simulink model "npc_controller"  (R2022a)
settings: Solver=FixedStepDiscrete  StartTime=0.0  StopTime=20  RelTol=1e-3  EnableMultiTasking=on
undefined symbols (not defined in the file): CAN_O_INT, CANA_BASE, Down, GPTRIP1SEL, GPTRIP2SEL, GPTRIP3SEL, Tsw, TZ1, TZ2, TZ3, Up, V2G_en
libraries: simulink x171, hdlsllib x90, c2802xlib x46, c2837xDlib x19, c280xlib x12, canmsglib x9, c2838xlib x8, idelinklib_common x5, c2806xlib x2, slpidlib x2, c28004xlib x2, c281xlib x2
(part 13 of 55)

== system npc_controller/IDLE_AND_TIMER/codegen/IDLE ==
  note: Note: GPIO6 J8.80
  note: Note: change to function call
  function : TriggerPort  TriggerType=function-call  VariantControl=Variant
  Function-Call Generator1 : simulink/Ports & Subsystems/Function-Call Generator  sample_time=-1  numberOfIterations=1  DisallowWideOutput=off
  Function-Call Split1 : FunctionCallSplit  NumOutputPorts=2
  Function-Call Split2 : FunctionCallSplit  NumOutputPorts=2
  Function-Call Split3 : FunctionCallSplit  NumOutputPorts=2
  GPIO6_HIGH : Subsystem  Commented=on
      settings: RTWSystemCode=Inline
  GPIO6_LOW : Subsystem  Commented=on
      settings: RTWSystemCode=Inline
  cnt_idle : Subsystem  TreatAsAtomicUnit=on
      settings: RTWSystemCode=Inline
  idle_task : Subsystem  TreatAsAtomicUnit=on
      settings: RTWSystemCode=Inline
  idle_task1 : Subsystem  Commented=on  TreatAsAtomicUnit=on
      settings: RTWSystemCode=Inline
  wires:
  Function-Call Split1/1 -> idle_task/Trigger
  Function-Call Split1/2 -> Function-Call Split2/1
  Function-Call Generator1/1 -> Function-Call Split3/1
  Function-Call Split3/1 -> GPIO6_HIGH/Trigger
  Function-Call Split3/2 -> Function-Call Split1/1
  Function-Call Split2/1 -> cnt_idle/Trigger
  Function-Call Split2/2 -> GPIO6_LOW/Trigger

== system npc_controller/IDLE_AND_TIMER/codegen/INITIALIZATION ==
  Function-Call Generator1 : simulink/Ports & Subsystems/Function-Call Generator  sample_time=-1  numberOfIterations=1  DisallowWideOutput=off
  Function-Call Split{1..3,5} (4 alike) : FunctionCallSplit  NumOutputPorts=2
  clb : Subsystem  Commented=on  TreatAsAtomicUnit=on
      settings: RTWSystemCode=Inline
  cmpss : Subsystem  TreatAsAtomicUnit=on
      settings: RTWSystemCode=Inline
  epwm : Subsystem  TreatAsAtomicUnit=on
      settings: RTWSystemCode=Inline
  epwm1 : Subsystem  Commented=on  TreatAsAtomicUnit=on
      settings: RTWSystemCode=Inline
  orps&relay : Subsystem  TreatAsAtomicUnit=on
      settings: RTWSystemCode=Inline
  outputxbar : Subsystem  Commented=on  TreatAsAtomicUnit=on
      settings: RTWSystemCode=Inline
  wires:
  Function-Call Generator1/1 -> Function-Call Split1/1
  Function-Call Split5/1 -> cmpss/Trigger
  Function-Call Split2/2 -> clb/Trigger
  Function-Call Split3/2 -> Function-Call Split5/1
  Function-Call Split2/1 -> outputxbar/Trigger
  Function-Call Split5/2 -> Function-Call Split2/1
  Function-Call Split3/1 -> orps&relay/Trigger
  Function-Call Split1/2 -> Function-Call Split3/1
  Function-Call Split1/1 -> epwm/Trigger

== system npc_controller/IDLE_AND_TIMER/codegen/TIMER_100MS ==
  note: Note: launchpad CANA, 32, 33
  note: Note:
      | Byte0 - func ID
      | Byte1 - MSB
      | Byte2 - LSB
  CAN Pack1 : canmsglib/CAN Pack  MsgList=(none)  MsgName=CAN Msg  MsgIDType=Standard (11-bit identifier)  MsgIdentifier=2  MsgLength=8  Remote=off  ApplyMinMax=off  BusOutput=off  SignalInfo={}
      settings: SourceProductBaseCode=ME,VN  DataFormat=raw data
  contstruct_can_msg : Subsystem
  eCAN Transmit : c280xlib/eCAN Transmit  chipFamily=C280x  useModule=eCAN_B  mailboxNo=1  messageID=bin2dec('111000111')  messageType=Standard (11-bit identifier)  enableBlockingMode=off  postInterrupt=off  interruptLine=0
      settings: SourceProductBaseCode=TIC2000
  get_func_id_data : Subsystem
  incr_cnt : Subsystem
  wires:
  CAN Pack1/1 -> eCAN Transmit/1
  contstruct_can_msg/1(can_msg) -> CAN Pack1/1
  get_func_id_data/2(data) -> contstruct_can_msg/2(data)
  get_func_id_data/1(func_id) -> contstruct_can_msg/1(func_id)

== system npc_controller/IDLE_AND_TIMER/codegen/TIMER_1MS ==
  note: 1) Add Subsystem or Model blocks as valid variant choices.
      | 2) You cannot connect blocks at this level. At simulation, connectivity is automatically
      | determined, based on the active variant and port name matching.
  codegen : Subsystem  VariantControl=sim_en==0
  sim : Subsystem  VariantControl=sim_en==1

== system npc_controller/IDLE_AND_TIMER/codegen/u32 Data to 2xu16 ==
  u32 Data : Inport
  Bit Shift : hdlsllib/Logic and Bit Operations/Bit Shift  mode=Shift Right Logical  N=8
  Bitwise AND : simulink/Logic and Bit Operations/Bitwise Operator  logicop=AND  UseBitMask=on  BitMask=bin2dec('00000000000000001111111111111111')  BitMaskRealWorld=Stored Integer
  Bitwise AND1 : simulink/Logic and Bit Operations/Bitwise Operator  logicop=AND  UseBitMask=on  BitMask=hex2dec('FFFF0000')  BitMaskRealWorld=Stored Integer
  Data Type Conversion : DataTypeConversion  OutDataTypeStr=uint16  SaturateOnIntegerOverflow=off  RndMeth=Floor
  Data Type Conversion1 : DataTypeConversion  OutDataTypeStr=uint16  SaturateOnIntegerOverflow=off  RndMeth=Floor
  u16Lsb : Outport
  u16Msb : Outport  Port=2
  wires:
  u32 Data/1 -> Bitwise AND1/1, Bitwise AND/1
  Bit Shift/1 -> Data Type Conversion1/1
  Bitwise AND/1 -> Data Type Conversion/1
  Data Type Conversion1/1 -> u16Msb/1
  Bitwise AND1/1 -> Bit Shift/1
  Data Type Conversion/1 -> u16Lsb/1

== system npc_controller/CONTROL/CONTROL/false/CLA_CONTROL ==
  va : Inport  OutDataTypeStr=single
  vb : Inport  Port=2  OutDataTypeStr=single
  vc : Inport  Port=3  OutDataTypeStr=single
  ia : Inport  Port=4  OutDataTypeStr=single
  ib : Inport  Port=5  OutDataTypeStr=single
  ic : Inport  Port=6  OutDataTypeStr=single
  vbulk : Inport  Port=7  OutDataTypeStr=single
  vmid : Inport  Port=8  OutDataTypeStr=single
  control_en : Inport  Port=9
  ref : Inport  Port=10
  angle : Inport  Port=11
  pol_pha : Inport  Port=12
  pol_phb : Inport  Port=13
  pol_phc : Inport  Port=14
  pha_en1 : Inport  Port=15
  phb_en1 : Inport  Port=16
  phc_en1 : Inport  Port=17
  pfc_ok2 : Inport  Port=18  OutDataTypeStr=boolean
  Trigger : TriggerPort  TriggerType=function-call  VariantControl=Variant  PortDimensions=1
  CONTROL : Subsystem
      settings: RTWSystemCode=Inline
  Function-Call Generator : simulink/Ports & Subsystems/Function-Call Generator  sample_time=-1  numberOfIterations=1  DisallowWideOutput=off
  Function-Call Split1 : FunctionCallSplit  NumOutputPorts=2
  Function-Call Split2 : FunctionCallSplit  NumOutputPorts=2
  Function-Call Split3 : FunctionCallSplit  NumOutputPorts=2
  GPIO_HIGH : Subsystem
      settings: RTWSystemCode=Inline
  GPIO_LOW : Subsystem
      settings: RTWSystemCode=Inline
  INIT/RESET_CONTROL : Subsystem
  sim_cmp : Outport
  Vpk : Outport  Port=2
  vbal_coef : Outport  Port=3
  wires:
  va/1 -> CONTROL/1(adc_out)  "cpu2cla_van"
  vb/1 -> CONTROL/2(adc_out1)  "cpu2cla_vbn"
  vc/1 -> CONTROL/3(adc_out2)  "cpu2cla_vcn"
  ia/1 -> CONTROL/4(adc_out3)  "cpu2cla_ia"
  ib/1 -> CONTROL/5(adc_out4)  "cpu2cla_ib"
  ic/1 -> CONTROL/6(adc_out5)  "cpu2cla_ic"
  vbulk/1 -> CONTROL/7(adc_out6)  "cpu2cla_vbulk"
  vmid/1 -> CONTROL/8(adc_out7)  "cpu2cla_vmid"
  ref/1 -> CONTROL/9(ref)  "cpu2cla_ref"
  Function-Call Split1/2 -> Function-Call Split3/1
  Function-Call Generator/1 -> Function-Call Split1/1
  Function-Call Split2/1 -> CONTROL/Trigger
  Function-Call Split2/2 -> GPIO_LOW/Trigger
  Function-Call Split1/1 -> GPIO_HIGH/Trigger
  CONTROL/1(sim_cmp) -> sim_cmp/1
  control_en/1 -> INIT/RESET_CONTROL/1(control_en)  "cpu2cla_control_en"
  Function-Call Split3/2 -> Function-Call Split2/1
  Function-Call Split3/1 -> INIT/RESET_CONTROL/Trigger
  pol_pha/1 -> CONTROL/11(pol_pha)  "cpu2cla_pol_pha"
  pol_phb/1 -> CONTROL/12(pol_phb)  "cpu2cla_pol_phb"
  pol_phc/1 -> CONTROL/13(pol_phc)  "cpu2cla_pol_phc"
  angle/1 -> CONTROL/10(angle)  "cpu2cla_angle"
  pha_en1/1 -> INIT/RESET_CONTROL/2(pha_en1)  "cpu2cla_pha_en"
  phb_en1/1 -> INIT/RESET_CONTROL/3(phb_en1)  "cpu2cla_phb_en"
  phc_en1/1 -> INIT/RESET_CONTROL/4(phc_en1)  "cpu2cla_phc_en"
  CONTROL/3(Vpk) -> Vpk/1  "cpu2cla_Vpk"
  pfc_ok2/1 -> CONTROL/14(pfc_ok2)  "cpu2cla_pfc_ok2"
  CONTROL/2(vbal_coef) -> vbal_coef/1  "cla2cpu_vbal_coef"

== system npc_controller/CONTROL/GET_ADC/ADC/codegen ==
  note: Note:
      | A0 VCSB_AD J3.30
      | A1 T_MUX_AD J7.70
      | A2 ICSC_AD J3.29
      | A3 VSCC_AD J3.26
      | A4 ICSA_AD J7.69
      | A5 VCSA_AD J7.66
      |
      | 14 ICSB_AD J3.23
      | 15 VBIAS_AD J7.63
      |
      | B0 IPHASE_A_ADC XX
      | B1 ADC_DEBUG_1 XX
      | B2 IPHASE_B_ADC J3.28
      | B3 IPHASE_C_ADC J3.25
      | B4 VPFC_OUT_AD J7.68
      | B5 VPFC_MID_AD J7.65
      |
      | *Near grid is ics
  adc_in : Inport
  3Ph Sine Gen : Subsystem  Commented=on
  ADCA : Subsystem
  ADCC : Subsystem
  Bus Creator1 : BusCreator  Inputs=8  OutDataTypeStr=Bus: adc
  Bus Creator2 : BusCreator  Inputs=8  OutDataTypeStr=Bus: adc_rect
  Constant : Constant  Commented=on  Value=2048  OutDataTypeStr=single  SampleTime=-1
  Data Store Read : DataStoreRead  Commented=on  DataStoreName=adc_vbulk  IndexOptions=Index vector (dialog)  Indices=1  OutputSizes=1
  Data Store Read1 : DataStoreRead  Commented=on  DataStoreName=adc_vmid  IndexOptions=Index vector (dialog)  Indices=1  OutputSizes=1
  Data Store Write7 : DataStoreWrite  Commented=on  DataStoreName=adc_vtop  IndexOptions=Index vector (dialog)  Indices=1  OutputSizes=1
  Function-Call Generator : simulink/Ports & Subsystems/Function-Call Generator  sample_time=-1  numberOfIterations=1  DisallowWideOutput=off
  Function-Call Split2 : FunctionCallSplit  NumOutputPorts=2
  Gain1 : Gain  Commented=on  Gain=2  ParamDataTypeStr=single  OutDataTypeStr=single
  Gain9 : Gain  Commented=on  Gain=2  ParamDataTypeStr=single  OutDataTypeStr=single
  IIR Filter7 : Subsystem  Commented=on
  Memory Copy : idelinklib_common/Memory Copy  Commented=on  copyFrom=Specified source code symbol  copyFromAddressSource=Specify via dialog  copyFromAddress=hex2dec('00001000')  copyFromSrcCode=&EPwm8Regs.CMPA.bit.CMPA  dataTypeFrom=uint16  dataDimensionFrom=1  useOffsetFrom=off  offsetFromSrc=Specify via dialog  offsetFrom=0  strideFrom=1  copyTo=Output port  copyToAddressSource=Specify via dialog  copyToAddress=hex2dec('00002000')  copyToSrcCode=myVariableDst  dataTypeTo=uint16  useOffsetTo=off  offsetToSrc=Specify via dialog  offsetTo=0  strideTo=1  sampleTime=inf  useInitValue=off  initValueSrc=Specify constant value  initValue=1  initValueSrcCode=myInitValueVariable  useAsMask=off  maskOperator=bitwise AND  useTermValue=off  termValue=1  isRealtimeEnabled=off  emitCCBeforeWrite=off  CCBeforeWrite=/* Custom Code Before Write*/  emitCCAfterWrite=off  CCAfterWrite=/* Custom Code After Write*/  useDMACopy=off  enableBlockingMode=off
      settings: SourceProductBaseCode=ME
  Memory Copy1 : idelinklib_common/Memory Copy  Commented=on  copyFrom=Specified source code symbol  copyFromAddressSource=Specify via dialog  copyFromAddress=hex2dec('00001000')  copyFromSrcCode=&EPwm2Regs.CMPB.bit.CMPB  dataTypeFrom=uint16  dataDimensionFrom=1  useOffsetFrom=off  offsetFromSrc=Specify via dialog  offsetFrom=0  strideFrom=1  copyTo=Output port  copyToAddressSource=Specify via dialog  copyToAddress=hex2dec('00002000')  copyToSrcCode=myVariableDst  dataTypeTo=uint16  useOffsetTo=off  offsetToSrc=Specify via dialog  offsetTo=0  strideTo=1  sampleTime=inf  useInitValue=off  initValueSrc=Specify constant value  initValue=1  initValueSrcCode=myInitValueVariable  useAsMask=off  maskOperator=bitwise AND  useTermValue=off  termValue=1  isRealtimeEnabled=off  emitCCBeforeWrite=off  CCBeforeWrite=/* Custom Code Before Write*/  emitCCAfterWrite=off  CCAfterWrite=/* Custom Code After Write*/  useDMACopy=off  enableBlockingMode=off
      settings: SourceProductBaseCode=ME
  Subsystem : Subsystem
  Subsystem1 : Subsystem
  Subsystem2 : Subsystem
  Subsystem3 : Subsystem
  Subsystem4 : Subsystem
  Subsystem5 : Subsystem
  Subsystem6 : Subsystem
  Subsystem7 : Subsystem
  Subsystem8 : Subsystem
  Subtract : Sum  Commented=on  Inputs=+-
  Sum : Sum  Commented=on  Inputs=|++
  adc_out : Outport
  adc_rect : Outport  Port=2
  wires:
  Data Store Read/1 -> Subtract/1
  Data Store Read1/1 -> Subtract/2
  Subtract/1 -> Data Store Write7/1
  [ic] -> Bus Creator1/6  "ic"
  [vmid] -> Bus Creator1/8  "vmid"
  [vbulk] -> Bus Creator1/7  "vbulk"
  Bus Creator1/1 -> adc_out/1  "vbulk"
  [ib] -> Bus Creator1/5  "ib"
  [ia] -> Bus Creator1/4  "ia"
  [ia] -> Subsystem3/1(adc)  "ia"
  [va] -> Subsystem/1(adc)  "va"
  [ic] -> Subsystem5/1(adc)  "ic"
  [vb] -> Subsystem1/1(adc)  "vb"
  [vmid] -> Bus Creator2/8  "vmid"
  [vc] -> Subsystem2/1(adc)  "vc"
  Subsystem5/1(adc_rect) -> Bus Creator2/6  "ic"
  [ib] -> Subsystem4/1(adc)  "ib"
  Subsystem4/1(adc_rect) -> Bus Creator2/5  "ib"
  Subsystem3/1(adc_rect) -> Bus Creator2/4  "ia"
  [vbulk] -> Bus Creator2/7  "vbulk"
  Bus Creator2/1 -> adc_rect/1
  Function-Call Split2/1 -> ADCA/Trigger
  Function-Call Generator/1 -> Function-Call Split2/1
  ADCA/1(vb) -> [vb]
  ADCA/4(ia) -> [ia]
  ADCA/3(vc) -> [vc]
  ADCA/2(ic) -> [ic]
  ADCA/5(va) -> [va]
  ADCA/6(ib) -> [ib]
  ADCC/4(vbulk) -> [vbulk]
  ADCC/5(vmid) -> [vmid]
  Function-Call Split2/2 -> ADCC/Trigger
  ADCC/3(iphasec) -> [iphasec]
  ADCC/2(iphaseb) -> [iphaseb]
  ADCC/1(iphasea) -> [iphasea]
  [iphasec] -> Subsystem8/1(adc)  "vc"
  [iphaseb] -> Subsystem7/1(adc)  "vb"
  [iphasea] -> Subsystem6/1(adc)  "va"
  3Ph Sine Gen/2(sine_b) -> Sum/1  "vb"
  Memory Copy/1 -> Gain9/1
  Gain9/1 -> ?
  Memory Copy1/1 -> Gain1/1
  Gain1/1 -> ?
  Sum/1 -> ?
  Constant/1 -> Sum/2
  [va] -> Bus Creator1/1  "va"
  [vb] -> Bus Creator1/2  "vb"
  [vc] -> Bus Creator1/3  "vc"
  Subsystem/1(adc_rect) -> Bus Creator2/1  "va"
  Subsystem1/1(adc_rect) -> Bus Creator2/2  "vb"
  Subsystem2/1(adc_rect) -> Bus Creator2/3  "vc"

== system npc_controller/CONTROL/GET_ADC/ADC/sim ==
  note: Notes:
      | vac_adc = vac_actual*0.00264706+1.65
      | iac_adc = iac_actual*0.02+1.65
      | vbulk_adc = vbulk_actual*3.49e-3
      | vmid_adc = vmid_acutal*3.49e-3
  note: Note:
      | Vmid         C2
      | Vbulk        A5
      |
      | Va            A2/B6
      | Vb            B0
      | Vc            C0
      |
      | Ia             A3
      | Ib             A10/B1, C10
      | Ic             C1
  note: since the current sense in hardware is -ve
  adc_in : Inport
  Bus Creator1 : BusCreator  Inputs=8  OutDataTypeStr=Bus: adc
  Bus Creator2 : BusCreator  Inputs=8  OutDataTypeStr=Bus: adc_rect
  Cast To Single : DataTypeConversion  OutDataTypeStr=single  SaturateOnIntegerOverflow=off  RndMeth=Floor
  Cast To Single1 : DataTypeConversion  OutDataTypeStr=single  SaturateOnIntegerOverflow=off  RndMeth=Floor
  Data Store Read : DataStoreRead  DataStoreName=adc_offset_vc  IndexOptions=Index vector (dialog)  Indices=1  OutputSizes=1
  Data Store Read1 : DataStoreRead  DataStoreName=adc_offset_ic  IndexOptions=Index vector (dialog)  Indices=1  OutputSizes=1
  Data Store Read2 : DataStoreRead  DataStoreName=adc_offset_vb  IndexOptions=Index vector (dialog)  Indices=1  OutputSizes=1
  Data Store Read4 : DataStoreRead  DataStoreName=adc_offset_va  IndexOptions=Index vector (dialog)  Indices=1  OutputSizes=1
  Data Store Read6 : DataStoreRead  DataStoreName=adc_offset_ia  IndexOptions=Index vector (dialog)  Indices=1  OutputSizes=1
  Data Store Read7 : DataStoreRead  DataStoreName=adc_offset_ib  IndexOptions=Index vector (dialog)  Indices=1  OutputSizes=1
  Demux : Demux  Outputs=8
  IIR Filter3 : Subsystem  Commented=on
  IIR Filter5 : Subsystem  Commented=on
  IIR Filter8 : Subsystem  Commented=on
  Scope2 : Scope
  Scope3 : Scope
  Subsystem : Subsystem
  Subsystem1 : Subsystem
  Subsystem2 : Subsystem
  Subsystem3 : Subsystem
  Subsystem4 : Subsystem
  Subsystem5 : Subsystem
  vabc{1..6} (6 alike) : Sum  Inputs=|+-  AccumDataTypeStr=single  OutDataTypeStr=single
  adc_out : Outport
  adc_rect : Outport  Port=2
  wires:
  adc_in/1 -> Demux/1
  Demux/7 -> Cast To Single/1
  Data Store Read6/1 -> vabc2/2
  Demux/4 -> vabc2/1
  vabc2/1 -> [ia]
  Bus Creator1/1 -> adc_out/1  "vbulk"
  Demux/6 -> vabc6/1
  Data Store Read2/1 -> vabc1/2
  Data Store Read1/1 -> Scope3/1, vabc6/2
  Data Store Read7/1 -> vabc5/2
  Demux/5 -> vabc5/1
  Demux/2 -> vabc1/1
  vabc3/1 -> [va]
  Data Store Read/1 -> Scope2/1, vabc4/2
  Data Store Read4/1 -> vabc3/2
  vabc1/1 -> [vb]
  vabc5/1 -> [ib]
  Demux/3 -> vabc4/1
  Demux/1 -> vabc3/1  "va"
  Demux/8 -> Cast To Single1/1  "vmid"
  [vb] -> Bus Creator1/2  "vb"
  [vc] -> Bus Creator1/3  "vc"
  [ia] -> Bus Creator1/4  "ia"
  [ib] -> Bus Creator1/5  "ib"
  [ic] -> Bus Creator1/6  "ic"
  [va] -> Bus Creator1/1  "va"
  [vbulk] -> Bus Creator1/7  "vbulk"
  [vmid] -> Bus Creator1/8  "vmid"
  Subsystem/1(adc_rect) -> Bus Creator2/1  "va"
  Subsystem1/1(adc_rect) -> Bus Creator2/2  "vb"
  Subsystem3/1(adc_rect) -> Bus Creator2/4  "ia"
  Subsystem4/1(adc_rect) -> Bus Creator2/5  "ib"
  Bus Creator2/1 -> adc_rect/1  "vbulk"
  [va] -> Subsystem/1(adc)  "va"
  [vb] -> Subsystem1/1(adc)  "vb"
  [vc] -> Subsystem2/1(adc)  "vc"
  [ia] -> Subsystem3/1(adc)  "ia"
  [ib] -> Subsystem4/1(adc)  "ib"
  [ic] -> Subsystem5/1(adc)  "ic"
  [vmid] -> Bus Creator2/8  "vmid"
  [vbulk] -> Bus Creator2/7  "vbulk"
  Subsystem2/1(adc_rect) -> Bus Creator2/3  "vc"
  Subsystem5/1(adc_rect) -> Bus Creator2/6  "ic"
  vabc4/1 -> [vc]  "va"
  vabc6/1 -> [ic]  "va"
  Cast To Single/1 -> [vbulk]
  Cast To Single1/1 -> [vmid]

== system npc_controller/CONTROL/POLARITY/PLL_Block1/SRF_PLL ==
  Vabc : Inport
  Demux1 : Demux  Outputs=3
  Gain : Gain  Commented=on  Gain=1/(2*pi)
  Integrator : Subsystem
  Memory : Memory  InheritSampleTime=on  LinearizeAsDelay=on
  PI : Subsystem
  Subsystem1 : Subsystem  Commented=on
  Sum1 : Sum  Inputs=|++  AccumDataTypeStr=single  OutDataTypeStr=single
  abc to dq : Subsystem
  f0 : Constant  Value=2*pi*50  OutDataTypeStr=fixdt('single', 'DataTypeOverride', 'Off')
  SinVal : Outport  VectorParamsAs1DForOutWhenUnconnected=off
  CosVal : Outport  Port=2  VectorParamsAs1DForOutWhenUnconnected=off
  theta : Outport  Port=3  OutDataTypeStr=single  VectorParamsAs1DForOutWhenUnconnected=off
  wires:
  Vabc/1 -> Demux1/1
  Memory/1 -> abc to dq/4(wt)
  Integrator/1(wt) -> Memory/1, theta/1
  abc to dq/1(q) -> PI/1(Vq)
  f0/1 -> Sum1/2
  Gain/1 -> Subsystem1/1(x[n])  "Freq_Unf"
  PI/1(PI Out) -> Sum1/1
  Sum1/1 -> Gain/1, Integrator/1(PI Out)
  Demux1/1 -> abc to dq/1(a)
  Demux1/2 -> abc to dq/2(b)
  Demux1/3 -> abc to dq/3(c)

== system npc_controller/CONTROL/POLARITY/PLL_Block1/Subsystem ==
  In1 : Inport
  Cast To Single : DataTypeConversion  OutDataTypeStr=single  SaturateOnIntegerOverflow=off  RndMeth=Floor
  Constant2 : Constant  Value=0
  GreaterThan1 : RelationalOperator  Operator=>  OutDataTypeStr=boolean  RndMeth=Simplest  InputSameDT=off
  Initialize at Zero Crossing : Subsystem  TreatAsAtomicUnit=on
  Out1 : Outport
  wires:
  GreaterThan1/1 -> Initialize at Zero Crossing/Trigger, Initialize at Zero Crossing/1(In1)
  Constant2/1 -> GreaterThan1/2
  Initialize at Zero Crossing/1(Out1) -> Cast To Single/1
  In1/1 -> GreaterThan1/1
  Cast To Single/1 -> Out1/1

== system npc_controller/CONTROL/STATE-MACHINE/CPU_CONTROL_100_A2_precharge_pfc_ok2/configFutDis/System Outputs1 ==

== system npc_controller/CONTROL/STATE-MACHINE/CPU_CONTROL_100_A2_precharge_pfc_ok2/configFutDis/System Outputs2 ==

== system npc_controller/CONTROL/STATE-MACHINE/CPU_CONTROL_100_A2_precharge_pfc_ok2/configFutEn/System Outputs1 ==

== system npc_controller/CONTROL/STATE-MACHINE/CPU_CONTROL_100_A2_precharge_pfc_ok2/configFutEn/System Outputs2 ==

== system npc_controller/CONTROL/STATE-MACHINE/CPU_CONTROL_100_A2_precharge_pfc_ok2/configFutEn/System Outputs3 ==

== system npc_controller/CONTROL/STATE-MACHINE/CPU_CONTROL_100_A2_precharge_pfc_ok2/configGrid/FORCE_TZ ==
  note: 0 - Three phase
      | 1 - Single phase
  In1 : Inport
  sinlgeph_config : Inport  Port=2
  Trigger : TriggerPort  TriggerType=function-call  VariantControl=(inherit)  PortDimensions=1
  1P : Subsystem  TreatAsAtomicUnit=on
  3P3W : Subsystem  TreatAsAtomicUnit=on
  If : If  IfExpression=u1 == 0
  wires:
  If/1 -> 3P3W/Action
  sinlgeph_config/1 -> 1P/1(sinlgeph_config)
  If/2 -> 1P/Action
  In1/1 -> If/1

== system npc_controller/CONTROL/STATE-MACHINE/CPU_CONTROL_100_A2_precharge_pfc_ok2/configGrid/RESET_TZ ==
  note: EALLOW;
      |
      | /*Disabled tripzone action*/
      | EPwm6Regs.TZCTL.bit.TZA = (uint16_T)(0b11); //do nothing
      | EPwm6Regs.TZCTL.bit.TZB = (uint16_T)(0b11);
      | EPwm7Regs.TZCTL.bit.TZA = (uint16_T)(0b11);
      | EPwm7Regs.TZCTL.bit.TZB = (uint16_T)(0b11);
      | EPwm8Regs.TZCTL.bit.TZA = (uint16_T)(0b11);
      | EPwm8Regs.TZCTL.bit.TZB = (uint16_T)(0b11);
      | EPwm9Regs.TZCTL.bit.TZA = (uint16_T)(0b11);
      | EPwm9Regs.TZCTL.bit.TZB = (uint16_T)(0b11);
      | EPwm10Regs.TZCTL.bit.TZA = (uint16_T)(0b11);
      | EPwm10Regs.TZCTL.bit.TZB = (uint16_T)(0b11);
      | EPwm11Regs.TZCTL.bit.TZA = (uint16_T)(0b11);
      | EPwm11Regs.TZCTL.bit.TZB = (uint16_T)(0b11);
      |
      | /*Clear grouped OST TZ flags*/
      | EPwm6Regs.TZCLR.bit.OST = 0b1; //clear trip
      | EPwm7Regs.TZCLR.bit.OST = 0b1;
      | EPwm8Regs.TZCLR.bit.OST = 0b1;
      | EPwm9Regs.TZCLR.bit.OST = 0b1;
      | EPwm10Regs.TZCLR.bit.OST = 0b1;
      | EPwm11Regs.TZCLR.bit.OST = 0b1;
      |
      | /*Clear individual OST TZ flags*/
      | EPwm6Regs.TZOSTCLR.bit.OST1 = 0b1; //clear trip
      | EPwm6Regs.TZOSTCLR.bit.OST2 = 0b1;
      | EPwm7Regs.TZOSTCLR.bit.OST1 = 0b1;
      | EPwm7Regs.TZOSTCLR.bit.OST2 = 0b1;
      | EPwm8Regs.TZOSTCLR.bit.OST1 = 0b1;
      | EPwm8Regs.TZOSTCLR.bit.OST2 = 0b1;
      | EPwm9Regs.TZOSTCLR.bit.OST1 = 0b1;
      | EPwm9Regs.TZOSTCLR.bit.OST2 = 0b1;
      | EPwm10Regs.TZOSTCLR.bit.OST1 = 0b1;
      | EPwm10Regs.TZOSTCLR.bit.OST2 = 0b1;
      | EPwm11Regs.TZOSTCLR.bit.OST1 = 0b1;
      | EPwm11Regs.TZOSTCLR.bit.OST2 = 0b1;
      |
      | /*Enable tripzone action*/
      | EPwm6Regs.TZCTL.bit.TZA = (uint16_T)(0b10); //force to LOW
      | EPwm6Regs.TZCTL.bit.TZB = (uint16_T)(0b10);
      | EPwm7Regs.TZCTL.bit.TZA = (uint16_T)(0b10);
      | EPwm7Regs.TZCTL.bit.TZB = (uint16_T)(0b10);
      | EPwm8Regs.TZCTL.bit.TZA = (uint16_T)(0b10);
      | EPwm8Regs.TZCTL.bit.TZB = (uint16_T)(0b10);
      | EPwm9Regs.TZCTL.bit.TZA = (uint16_T)(0b10);
      | EPwm9Regs.TZCTL.bit.TZB = (uint16_T)(0b10);
      | EPwm10Regs.TZCTL.bit.TZA = (uint16_T)(0b10);
      | EPwm10Regs.TZCTL.bit.TZB = (uint16_T)(0b10);
      | EPwm11Regs.TZCTL.bit.TZA = (uint16_T)(0b10);
      | EPwm11Regs.TZCTL.bit.TZB = (uint16_T)(0b10);
      |
      | EDIS;
  note: Note:
      | TZCCTL
      | 0b00 - High impedance
      | 0b01 - Force to HIGH
      | 0b10 - Force to LOW
      | 0b11 - Do nothing
      |
      | AQCSFRC
      | 0b00 - disables forced PWM
      | 0b01 - forces PWM to LOW
      | 0b10 - forces PWM to  HIGH
      |
      | TZFRC.bit.OST
      | 0b0 - Do nothing
      | 0b1 - Force TZ
  Trigger : TriggerPort  TriggerType=function-call  VariantControl=(inherit)  PortDimensions=1
  System Outputs2 : Subsystem  mask(System Outputs){ShowInLibBrowser=0}
      mask prompts: ShowInLibBrowser "Simulink:masks:CustCodeMaskParam1_MP"
      settings: CopyFcn=cccopyfcn(gcb)  OpenFcn=ccopenfcn('System Outputs Function')
      mask Help: eval('feval(''rtwprivate'',''rtwhelpview'',''rtw_sys_outputs_block'')');
      mask Display: disp('System\nOutputs');

== system npc_controller/CONTROL/STATE-MACHINE/CPU_CONTROL_100_A2_precharge_pfc_ok2/detectPOSPhB/pos ==
  note: Note:
      | AQCSFRC
      | 0b00 - disables forced PWM
      | 0b01 - forces PWM to LOW
      | 0b10 - forces PWM to  HIGH
  note: Note:
      |
      | Function PWM # GPIO # LAUNCHPAD PIN #
      |
      | Synci EPWM1A GPIO0 J4.40
      | EPWM1B GPIO1 J4.39
      |
      | TZ GPIO62 XX
      |
      | a_s1 EPWM6B GPIO11 J8.75
      | a_s2 EPWM7B GPIO13 XX
      | a_s3 EPWM6A GPIO10 J8.76
      | a_s4 EPWM7A GPIO12 XX
      |
      | b_s1 EPWM8B GPIO15 J8.73
      | b_s2 EPWM9B GPIO17 XX
      | b_s3 EPWM8A GPIO14 J8.74
      | b_s4 EPWM9A GPIO16 J4.33
      |
      | c_s1 EPWM10B GPIO19 J1.3
      | c_s2 EPWM11B GPIO21 XX
      | c_s3 EPWM10A GPIO18 J1.4
      | c_s4 EPWM11A GPIO20 XX
  note: EPwm8Regs.AQCSFRC.bit.CSFB = (uint16_T)(0b01);
      | EPwm9Regs.AQCSFRC.bit.CSFB = (uint16_T)(0b10);
      | EPwm8Regs.AQCSFRC.bit.CSFA = (uint16_T)(0b00);
      | EPwm9Regs.AQCSFRC.bit.CSFA = (uint16_T)(0b01);
  Action Port : ActionPort  ActionPortLabel=elseif(u1 >= 16)
  Constant : Constant  OutDataTypeStr=uint8  SampleTime=-1
  System Outputs1 : Subsystem  mask(System Outputs){ShowInLibBrowser=0}
      mask prompts: ShowInLibBrowser "Simulink:masks:CustCodeMaskParam1_MP"
      settings: CopyFcn=cccopyfcn(gcb)  OpenFcn=ccopenfcn('System Outputs Function')
      mask Help: eval('feval(''rtwprivate'',''rtwhelpview'',''rtw_sys_outputs_block'')');
      mask Display: disp('System\nOutputs');
  pos : Outport
  wires:
  Constant/1 -> pos/1

== system npc_controller/CONTROL/STATE-MACHINE/CPU_CONTROL_100_A2_precharge_pfc_ok2/detectUvpOvp1/False ==
  Action Port : ActionPort
  Constant : Constant  Value=0  OutDataTypeStr=boolean  SampleTime=-1
  low : Outport
  wires:
  Constant/1 -> low/1

== system npc_controller/CONTROL/STATE-MACHINE/CPU_CONTROL_100_A2_precharge_pfc_ok2/detectUvpOvp1/True ==
  Action Port : ActionPort
  Constant1 : Constant  OutDataTypeStr=boolean  SampleTime=-1
  high : Outport
  wires:
  Constant1/1 -> high/1

== system npc_controller/CONTROL/STATE-MACHINE/CPU_CONTROL_100_A2_precharge_pfc_ok2/detectZCPhA/false ==
  Action Port : ActionPort  ActionPortLabel=else
  Constant1 : Constant  Value=0  OutDataTypeStr=boolean  SampleTime=-1
  ph_en_out : Outport
  wires:
  Constant1/1 -> ph_en_out/1

== system npc_controller/CONTROL/STATE-MACHINE/CPU_CONTROL_100_A2_precharge_pfc_ok2/detectZCPhA/true ==
  Action Port : ActionPort  ActionPortLabel="if((u1 > -5)  & (u1 < 5))"
  Constant : Constant  OutDataTypeStr=boolean  SampleTime=-1
  ph_en : Outport
  wires:
  Constant/1 -> ph_en/1

== system npc_controller/CONTROL/STATE-MACHINE/CPU_CONTROL_100_A2_precharge_pfc_ok2/detectZCPhB/false ==
  Action Port : ActionPort  ActionPortLabel=else
  Constant1 : Constant  Value=0  OutDataTypeStr=boolean  SampleTime=-1
  ph_en_out : Outport
  wires:
  Constant1/1 -> ph_en_out/1

== system npc_controller/CONTROL/STATE-MACHINE/CPU_CONTROL_100_A2_precharge_pfc_ok2/detectZCPhB/true ==
  Action Port : ActionPort  ActionPortLabel="if((u1 > -5)  & (u1 < 5))"
  Constant : Constant  OutDataTypeStr=boolean  SampleTime=-1
  ph_en : Outport
  wires:
  Constant/1 -> ph_en/1

== system npc_controller/CONTROL/STATE-MACHINE/CPU_CONTROL_100_A2_precharge_pfc_ok2/detectZCPhC/false ==
  Action Port : ActionPort  ActionPortLabel=else
  Constant1 : Constant  Value=0  OutDataTypeStr=boolean  SampleTime=-1
  ph_en_out : Outport
  wires:
  Constant1/1 -> ph_en_out/1

== system npc_controller/CONTROL/STATE-MACHINE/CPU_CONTROL_100_A2_precharge_pfc_ok2/detectZCPhC/true ==
  Action Port : ActionPort  ActionPortLabel="if((u1 > -5)  & (u1 < 5))"
  Constant : Constant  OutDataTypeStr=boolean  SampleTime=-1
  ph_en : Outport
  wires:
  Constant/1 -> ph_en/1

== system npc_controller/CONTROL/STATE-MACHINE/CPU_CONTROL_100_A2_precharge_pfc_ok2/disDigCmpMode/System Outputs2 ==

== system npc_controller/CONTROL/STATE-MACHINE/CPU_CONTROL_100_A2_precharge_pfc_ok2/disablePwm/System Outputs ==

== system npc_controller/CONTROL/STATE-MACHINE/CPU_CONTROL_100_A2_precharge_pfc_ok2/enDigCmpMode/System Outputs2 ==

== system npc_controller/CONTROL/STATE-MACHINE/CPU_CONTROL_100_A2_precharge_pfc_ok2/updateCalib/cnt ==
  cnt_calib : Inport  OutDataTypeStr=uint16
  van : Inport  Port=2  OutDataTypeStr=single  PortDimensions=1
  vbn : Inport  Port=3  OutDataTypeStr=single  PortDimensions=1
  vcn : Inport  Port=4  OutDataTypeStr=single  PortDimensions=1
  ia : Inport  Port=5  OutDataTypeStr=single  PortDimensions=1
  ib : Inport  Port=6  OutDataTypeStr=single  PortDimensions=1
  ic : Inport  Port=7  OutDataTypeStr=single  PortDimensions=1
  Action Port : ActionPort  ActionPortLabel=else
  Add : Sum  AccumDataTypeStr=uint16  OutDataTypeStr=uint16
  Constant : Constant  OutDataTypeStr=uint16  SampleTime=-1
  Constant1 : Constant  Value=0  OutDataTypeStr=boolean  SampleTime=-1
  Data Store Write : DataStoreWrite  DataStoreName=adc_offset_ib_tmp  IndexOptions=Index vector (dialog)  Indices=1  OutputSizes=1
  Data Store Write1 : DataStoreWrite  DataStoreName=adc_offset_ic_tmp  IndexOptions=Index vector (dialog)  Indices=1  OutputSizes=1
  Data Store Write2 : DataStoreWrite  DataStoreName=cnt_calib  IndexOptions=Index vector (dialog)  Indices=1  OutputSizes=1
  Data Store Write3 : DataStoreWrite  DataStoreName=adc_offset_vc_tmp  IndexOptions=Index vector (dialog)  Indices=1  OutputSizes=1
  Data Store Write4 : DataStoreWrite  DataStoreName=adc_offset_ia_tmp  IndexOptions=Index vector (dialog)  Indices=1  OutputSizes=1
  Data Store Write5 : DataStoreWrite  DataStoreName=adc_offset_va_tmp  IndexOptions=Index vector (dialog)  Indices=1  OutputSizes=1
  Data Store Write6 : DataStoreWrite  DataStoreName=adc_offset_vb_tmp  IndexOptions=Index vector (dialog)  Indices=1  OutputSizes=1
  IIR Filter2 : Subsystem  Commented=on
  Subsystem1 : Subsystem
  Subsystem2 : Subsystem
  Subsystem3 : Subsystem
  Subsystem4 : Subsystem
  Subsystem5 : Subsystem
  Subsystem6 : Subsystem
  calib_ok : Outport
  wires:
  cnt_calib/1 -> Add/1
  Add/1 -> Data Store Write2/1
  Constant1/1 -> calib_ok/1
  Subsystem2/1(average) -> Data Store Write/1  "va"
  Constant/1 -> Add/2
  Subsystem1/1(average) -> Data Store Write1/1  "va"
  Subsystem3/1(average) -> Data Store Write4/1  "va"
  Subsystem4/1(average) -> Data Store Write3/1  "va"
  Subsystem6/1(average) -> Data Store Write5/1  "va"
  van/1 -> Subsystem6/1(sample)
  Subsystem5/1(average) -> Data Store Write6/1  "va"
  vcn/1 -> Subsystem4/1(sample)
  vbn/1 -> Subsystem5/1(sample)
  ia/1 -> Subsystem3/1(sample)
  ic/1 -> Subsystem1/1(sample)
  ib/1 -> Subsystem2/1(sample)

== system npc_controller/CONTROL/STATE-MACHINE/CPU_CONTROL_100_A2_precharge_pfc_ok2/updateCalib/done ==
  Action Port : ActionPort  ActionPortLabel=if(u1 > 65000)
  AUTO-CALIB_DONE : Subsystem
  CLEAR_FAULTS : Subsystem
  Function-Call Generator : simulink/Ports & Subsystems/Function-Call Generator  sample_time=-1  numberOfIterations=1  DisallowWideOutput=off
  Function-Call Split1 : FunctionCallSplit  NumOutputPorts=2
  Function-Call Split2 : FunctionCallSplit  NumOutputPorts=2
  RESET_TZ : Subsystem
  calib_ok : Outport
  wires:
  Function-Call Generator/1 -> Function-Call Split1/1
  Function-Call Split1/2 -> Function-Call Split2/1
  AUTO-CALIB_DONE/1(Out1) -> calib_ok/1
  Function-Call Split1/1 -> AUTO-CALIB_DONE/Trigger
  Function-Call Split2/1 -> RESET_TZ/Trigger
  Function-Call Split2/2 -> CLEAR_FAULTS/Trigger

== system npc_controller/CONTROL/STATE-MACHINE/CPU_CONTROL_100_A2_precharge_pfc_ok2/updatePll3p/PLL ==
  abc : Inport
  Demux : Demux  Commented=on  Outputs=3
  If1 : If  Commented=on  IfExpression=(u1 > 0)  ShowElse=off
  SRF_PLL : Subsystem
  Subsystem : Subsystem  Commented=on
  theta : Outport  OutDataTypeStr=single
  wires:
  SRF_PLL/3(theta) -> theta/1
  Subsystem/1(Out1) -> If1/1
  abc/1 -> SRF_PLL/1(Vabc), Demux/1
  Demux/1 -> Subsystem/1(In1)

== system npc_controller/CONTROL/STATE-MACHINE/CPU_CONTROL_100_A2_precharge_pfc_ok2/updateSequencePhA/pol_final1 ==
  vxn : Inport
  ix : Inport  Port=2
  Trigger : TriggerPort  TriggerType=function-call  VariantControl=(inherit)  PortDimensions=1
  If : If  NumInputs=2  IfExpression="((u1 == 1)  & (u2 == 2)) | ((u1 == 2)  & (u2 == 1))"
  Merge : Merge
  pol_vxn : Subsystem  TreatAsAtomicUnit=on
  prot : Subsystem  TreatAsAtomicUnit=on
  pol : Outport
  wires:
  ix/1 -> If/2
  vxn/1 -> pol_vxn/1(vxn), If/1
  Merge/1 -> pol/1
  If/2 -> pol_vxn/Action
  prot/1(Out1) -> Merge/1
  If/1 -> prot/Action
  pol_vxn/1(Out1) -> Merge/2

== system npc_controller/CONTROL/STATE-MACHINE/CPU_CONTROL_100_A2_precharge_pfc_ok2/updateSequencePhA/pol_ix1 ==
  note: 75dig -> 3iac
  ix : Inport
  Trigger : TriggerPort  TriggerType=function-call  VariantControl=(inherit)  PortDimensions=1
  If : If  IfExpression="(u1 > -8)  & (u1 < 8)"  ElseIfExpressions=u1 >= 8
  Merge : Merge  Inputs=3
  neg : Subsystem  TreatAsAtomicUnit=on
  pos : Subsystem  TreatAsAtomicUnit=on
  zero : Subsystem  TreatAsAtomicUnit=on
  pol_ix : Outport
  wires:
  ix/1 -> If/1
  If/1 -> zero/Action
  zero/1(Out1) -> Merge/1
  If/2 -> pos/Action
  If/3 -> neg/Action
  neg/1(Out1) -> Merge/3
  pos/1(Out1) -> Merge/2
  Merge/1 -> pol_ix/1

== system npc_controller/CONTROL/STATE-MACHINE/CPU_CONTROL_100_A2_precharge_pfc_ok2/updateSequencePhA/pol_vxn1 ==
  note: 16dig -> 5vac
  vxn : Inport
  Trigger : TriggerPort  TriggerType=function-call  VariantControl=(inherit)  PortDimensions=1
  If : If  IfExpression="(u1 > -16)  & (u1 < 16)"  ElseIfExpressions=u1 >= 16
  Merge : Merge  Inputs=3
  neg : Subsystem  TreatAsAtomicUnit=on
  pos : Subsystem  TreatAsAtomicUnit=on
  zero : Subsystem  TreatAsAtomicUnit=on
  pol_vxn : Outport
  wires:
  Merge/1 -> pol_vxn/1
  pos/1(Out1) -> Merge/2
  neg/1(Out1) -> Merge/3
  If/3 -> neg/Action
  If/2 -> pos/Action
  zero/1(Out1) -> Merge/1
  If/1 -> zero/Action
  vxn/1 -> If/1

== system npc_controller/CONTROL/STATE-MACHINE/CPU_CONTROL_100_A2_precharge_pfc_ok2/updateSequencePhB/pol_final1 ==
  vxn : Inport
  ix : Inport  Port=2
  Trigger : TriggerPort  TriggerType=function-call  VariantControl=(inherit)  PortDimensions=1
  If : If  NumInputs=2  IfExpression="((u1 == 1)  & (u2 == 2)) | ((u1 == 2)  & (u2 == 1))"
  Merge : Merge
  pol_vxn : Subsystem  TreatAsAtomicUnit=on
  prot : Subsystem  TreatAsAtomicUnit=on
  pol : Outport
  wires:
  ix/1 -> If/2
  vxn/1 -> pol_vxn/1(vxn), If/1
  Merge/1 -> pol/1
  If/2 -> pol_vxn/Action
  prot/1(Out1) -> Merge/1
  If/1 -> prot/Action
  pol_vxn/1(Out1) -> Merge/2

== system npc_controller/CONTROL/STATE-MACHINE/CPU_CONTROL_100_A2_precharge_pfc_ok2/updateSequencePhB/pol_ix1 ==
  note: 75dig -> 3iac
  ix : Inport
  Trigger : TriggerPort  TriggerType=function-call  VariantControl=(inherit)  PortDimensions=1
  If : If  IfExpression="(u1 > -8)  & (u1 < 8)"  ElseIfExpressions=u1 >= 8
  Merge : Merge  Inputs=3
  neg : Subsystem  TreatAsAtomicUnit=on
  pos : Subsystem  TreatAsAtomicUnit=on
  zero : Subsystem  TreatAsAtomicUnit=on
  pol_ix : Outport
  wires:
  ix/1 -> If/1
  If/1 -> zero/Action
  zero/1(Out1) -> Merge/1
  If/2 -> pos/Action
  If/3 -> neg/Action
  neg/1(Out1) -> Merge/3
  pos/1(Out1) -> Merge/2
  Merge/1 -> pol_ix/1

== system npc_controller/CONTROL/STATE-MACHINE/CPU_CONTROL_100_A2_precharge_pfc_ok2/updateSequencePhB/pol_vxn1 ==
  note: 16dig -> 5vac
  vxn : Inport
  Trigger : TriggerPort  TriggerType=function-call  VariantControl=(inherit)  PortDimensions=1
  If : If  IfExpression="(u1 > -16)  & (u1 < 16)"  ElseIfExpressions=u1 >= 16
  Merge : Merge  Inputs=3
  neg : Subsystem  TreatAsAtomicUnit=on
  pos : Subsystem  TreatAsAtomicUnit=on
  zero : Subsystem  TreatAsAtomicUnit=on
  pol_vxn : Outport
  wires:
  Merge/1 -> pol_vxn/1
  pos/1(Out1) -> Merge/2
  neg/1(Out1) -> Merge/3
  If/3 -> neg/Action
  If/2 -> pos/Action
  zero/1(Out1) -> Merge/1
  If/1 -> zero/Action
  vxn/1 -> If/1

== system npc_controller/CONTROL/STATE-MACHINE/CPU_CONTROL_100_A2_precharge_pfc_ok2/updateSequencePhC/pol_final1 ==
  vxn : Inport
  ix : Inport  Port=2
  Trigger : TriggerPort  TriggerType=function-call  VariantControl=(inherit)  PortDimensions=1
  If : If  NumInputs=2  IfExpression="((u1 == 1)  & (u2 == 2)) | ((u1 == 2)  & (u2 == 1))"
  Merge : Merge
  pol_vxn : Subsystem  TreatAsAtomicUnit=on
  prot : Subsystem  TreatAsAtomicUnit=on
  pol : Outport
  wires:
  ix/1 -> If/2
  vxn/1 -> pol_vxn/1(vxn), If/1
  Merge/1 -> pol/1
  If/2 -> pol_vxn/Action
  prot/1(Out1) -> Merge/1
  If/1 -> prot/Action
  pol_vxn/1(Out1) -> Merge/2

== system npc_controller/CONTROL/STATE-MACHINE/CPU_CONTROL_100_A2_precharge_pfc_ok2/updateSequencePhC/pol_ix1 ==
  note: 75dig -> 3iac
  ix : Inport
  Trigger : TriggerPort  TriggerType=function-call  VariantControl=(inherit)  PortDimensions=1
  If : If  IfExpression="(u1 > -8)  & (u1 < 8)"  ElseIfExpressions=u1 >= 8
  Merge : Merge  Inputs=3
  neg : Subsystem  TreatAsAtomicUnit=on
  pos : Subsystem  TreatAsAtomicUnit=on
  zero : Subsystem  TreatAsAtomicUnit=on
  pol_ix : Outport
  wires:
  ix/1 -> If/1
  If/1 -> zero/Action
  zero/1(Out1) -> Merge/1
  If/2 -> pos/Action
  If/3 -> neg/Action
  neg/1(Out1) -> Merge/3
  pos/1(Out1) -> Merge/2
  Merge/1 -> pol_ix/1

== system npc_controller/CONTROL/STATE-MACHINE/CPU_CONTROL_100_A2_precharge_pfc_ok2/updateSequencePhC/pol_vxn1 ==
  note: 16dig -> 5vac
  vxn : Inport
  Trigger : TriggerPort  TriggerType=function-call  VariantControl=(inherit)  PortDimensions=1
  If : If  IfExpression="(u1 > -16)  & (u1 < 16)"  ElseIfExpressions=u1 >= 16
  Merge : Merge  Inputs=3
  neg : Subsystem  TreatAsAtomicUnit=on
  pos : Subsystem  TreatAsAtomicUnit=on
  zero : Subsystem  TreatAsAtomicUnit=on
  pol_vxn : Outport
  wires:
  Merge/1 -> pol_vxn/1
  pos/1(Out1) -> Merge/2
  neg/1(Out1) -> Merge/3
  If/3 -> neg/Action
  If/2 -> pos/Action
  zero/1(Out1) -> Merge/1
  If/1 -> zero/Action
  vxn/1 -> If/1

== system npc_controller/CONTROL/STATE-MACHINE/CPU_CONTROL_100_inv/ClrCmpssTz/System Outputs1 ==

== system npc_controller/CONTROL/STATE-MACHINE/CPU_CONTROL_100_inv/ClrCmpssTz/System Outputs2 ==

== system npc_controller/CONTROL/STATE-MACHINE/CPU_CONTROL_100_inv/configFutDis/System Outputs1 ==

== system npc_controller/CONTROL/STATE-MACHINE/CPU_CONTROL_100_inv/configFutDis/System Outputs2 ==

== system npc_controller/CONTROL/STATE-MACHINE/CPU_CONTROL_100_inv/configFutEn/System Outputs1 ==

== system npc_controller/CONTROL/STATE-MACHINE/CPU_CONTROL_100_inv/configFutEn/System Outputs2 ==

== system npc_controller/CONTROL/STATE-MACHINE/CPU_CONTROL_100_inv/configFutEn/System Outputs3 ==

== system npc_controller/CONTROL/STATE-MACHINE/CPU_CONTROL_100_inv/configGrid/FORCE_TZ ==
  note: 0 - Three phase
      | 1 - Single phase
  In1 : Inport
  sinlgeph_config : Inport  Port=2
  Trigger : TriggerPort  TriggerType=function-call  VariantControl=(inherit)  PortDimensions=1
  1P : Subsystem  TreatAsAtomicUnit=on
  3P3W : Subsystem  TreatAsAtomicUnit=on
  If : If  IfExpression=u1 == 0
  wires:
  If/1 -> 3P3W/Action
  sinlgeph_config/1 -> 1P/1(sinlgeph_config)
  If/2 -> 1P/Action
  In1/1 -> If/1

== system npc_controller/CONTROL/STATE-MACHINE/CPU_CONTROL_100_inv/configGrid/RESET_TZ ==
  note: EALLOW;
      |
      | /*Disabled tripzone action*/
      | EPwm6Regs.TZCTL.bit.TZA = (uint16_T)(0b11); //do nothing
      | EPwm6Regs.TZCTL.bit.TZB = (uint16_T)(0b11);
      | EPwm7Regs.TZCTL.bit.TZA = (uint16_T)(0b11);
      | EPwm7Regs.TZCTL.bit.TZB = (uint16_T)(0b11);
      | EPwm8Regs.TZCTL.bit.TZA = (uint16_T)(0b11);
      | EPwm8Regs.TZCTL.bit.TZB = (uint16_T)(0b11);
      | EPwm9Regs.TZCTL.bit.TZA = (uint16_T)(0b11);
      | EPwm9Regs.TZCTL.bit.TZB = (uint16_T)(0b11);
      | EPwm10Regs.TZCTL.bit.TZA = (uint16_T)(0b11);
      | EPwm10Regs.TZCTL.bit.TZB = (uint16_T)(0b11);
      | EPwm11Regs.TZCTL.bit.TZA = (uint16_T)(0b11);
      | EPwm11Regs.TZCTL.bit.TZB = (uint16_T)(0b11);
      |
      | /*Clear grouped OST TZ flags*/
      | EPwm6Regs.TZCLR.bit.OST = 0b1; //clear trip
      | EPwm7Regs.TZCLR.bit.OST = 0b1;
      | EPwm8Regs.TZCLR.bit.OST = 0b1;
      | EPwm9Regs.TZCLR.bit.OST = 0b1;
      | EPwm10Regs.TZCLR.bit.OST = 0b1;
      | EPwm11Regs.TZCLR.bit.OST = 0b1;
      |
      | /*Clear individual OST TZ flags*/
      | EPwm6Regs.TZOSTCLR.bit.OST1 = 0b1; //clear trip
      | EPwm6Regs.TZOSTCLR.bit.OST2 = 0b1;
      | EPwm7Regs.TZOSTCLR.bit.OST1 = 0b1;
      | EPwm7Regs.TZOSTCLR.bit.OST2 = 0b1;
      | EPwm8Regs.TZOSTCLR.bit.OST1 = 0b1;
      | EPwm8Regs.TZOSTCLR.bit.OST2 = 0b1;
      | EPwm9Regs.TZOSTCLR.bit.OST1 = 0b1;
      | EPwm9Regs.TZOSTCLR.bit.OST2 = 0b1;
      | EPwm10Regs.TZOSTCLR.bit.OST1 = 0b1;
      | EPwm10Regs.TZOSTCLR.bit.OST2 = 0b1;
      | EPwm11Regs.TZOSTCLR.bit.OST1 = 0b1;
      | EPwm11Regs.TZOSTCLR.bit.OST2 = 0b1;
      |
      | /*Enable tripzone action*/
      | EPwm6Regs.TZCTL.bit.TZA = (uint16_T)(0b10); //force to LOW
      | EPwm6Regs.TZCTL.bit.TZB = (uint16_T)(0b10);
      | EPwm7Regs.TZCTL.bit.TZA = (uint16_T)(0b10);
      | EPwm7Regs.TZCTL.bit.TZB = (uint16_T)(0b10);
      | EPwm8Regs.TZCTL.bit.TZA = (uint16_T)(0b10);
      | EPwm8Regs.TZCTL.bit.TZB = (uint16_T)(0b10);
      | EPwm9Regs.TZCTL.bit.TZA = (uint16_T)(0b10);
      | EPwm9Regs.TZCTL.bit.TZB = (uint16_T)(0b10);
      | EPwm10Regs.TZCTL.bit.TZA = (uint16_T)(0b10);
      | EPwm10Regs.TZCTL.bit.TZB = (uint16_T)(0b10);
      | EPwm11Regs.TZCTL.bit.TZA = (uint16_T)(0b10);
      | EPwm11Regs.TZCTL.bit.TZB = (uint16_T)(0b10);
      |
      | EDIS;
  note: Note:
      | TZCCTL
      | 0b00 - High impedance
      | 0b01 - Force to HIGH
      | 0b10 - Force to LOW
      | 0b11 - Do nothing
      |
      | AQCSFRC
      | 0b00 - disables forced PWM
      | 0b01 - forces PWM to LOW
      | 0b10 - forces PWM to  HIGH
      |
      | TZFRC.bit.OST
      | 0b0 - Do nothing
      | 0b1 - Force TZ
  Trigger : TriggerPort  TriggerType=function-call  VariantControl=(inherit)  PortDimensions=1
  System Outputs2 : Subsystem  mask(System Outputs){ShowInLibBrowser=0}
      mask prompts: ShowInLibBrowser "Simulink:masks:CustCodeMaskParam1_MP"
      settings: CopyFcn=cccopyfcn(gcb)  OpenFcn=ccopenfcn('System Outputs Function')
      mask Help: eval('feval(''rtwprivate'',''rtwhelpview'',''rtw_sys_outputs_block'')');
      mask Display: disp('System\nOutputs');

== system npc_controller/CONTROL/STATE-MACHINE/CPU_CONTROL_100_inv/detectZCPhA/false ==
  Action Port : ActionPort
  Constant1 : Constant  Value=0  OutDataTypeStr=boolean  SampleTime=-1
  ph_en_out : Outport
  wires:
  Constant1/1 -> ph_en_out/1

== system npc_controller/CONTROL/STATE-MACHINE/CPU_CONTROL_100_inv/detectZCPhA/true ==
  Action Port : ActionPort
  Constant : Constant  OutDataTypeStr=boolean  SampleTime=-1
  ph_en : Outport
  wires:
  Constant/1 -> ph_en/1

== system npc_controller/CONTROL/STATE-MACHINE/CPU_CONTROL_100_inv/detectZCPhB/false ==
  Action Port : ActionPort
  Constant1 : Constant  Value=0  OutDataTypeStr=boolean  SampleTime=-1
  ph_en_out : Outport
  wires:
  Constant1/1 -> ph_en_out/1

== system npc_controller/CONTROL/STATE-MACHINE/CPU_CONTROL_100_inv/detectZCPhB/true ==
  Action Port : ActionPort
  Constant : Constant  OutDataTypeStr=boolean  SampleTime=-1
  ph_en : Outport
  wires:
  Constant/1 -> ph_en/1

== system npc_controller/CONTROL/STATE-MACHINE/CPU_CONTROL_100_inv/detectZCPhC/false ==
  Action Port : ActionPort
  Constant1 : Constant  Value=0  OutDataTypeStr=boolean  SampleTime=-1
  ph_en_out : Outport
  wires:
  Constant1/1 -> ph_en_out/1

== system npc_controller/CONTROL/STATE-MACHINE/CPU_CONTROL_100_inv/detectZCPhC/true ==
  Action Port : ActionPort
  Constant : Constant  OutDataTypeStr=boolean  SampleTime=-1
  ph_en : Outport
  wires:
  Constant/1 -> ph_en/1

== system npc_controller/CONTROL/STATE-MACHINE/CPU_CONTROL_100_inv/disCmpssTz/System Outputs1 ==

== system npc_controller/CONTROL/STATE-MACHINE/CPU_CONTROL_100_inv/disCmpssTz/System Outputs2 ==

== system npc_controller/CONTROL/STATE-MACHINE/CPU_CONTROL_100_inv/disablePwm/System Outputs ==

== system npc_controller/CONTROL/STATE-MACHINE/CPU_CONTROL_100_inv/readCmpssOcp/System Outputs1 ==

== system npc_controller/CONTROL/STATE-MACHINE/CPU_CONTROL_100_inv/updateCalib/cnt ==
  cnt_calib : Inport  OutDataTypeStr=uint16
  van : Inport  Port=2  OutDataTypeStr=single  PortDimensions=1
  vbn : Inport  Port=3  OutDataTypeStr=single  PortDimensions=1
  vcn : Inport  Port=4  OutDataTypeStr=single  PortDimensions=1
  ia : Inport  Port=5  OutDataTypeStr=single  PortDimensions=1
  ib : Inport  Port=6  OutDataTypeStr=single  PortDimensions=1
  ic : Inport  Port=7  OutDataTypeStr=single  PortDimensions=1
  Action Port : ActionPort
  Add : Sum  AccumDataTypeStr=uint16  OutDataTypeStr=uint16
  Constant : Constant  OutDataTypeStr=uint16  SampleTime=-1
  Constant1 : Constant  Value=0  OutDataTypeStr=boolean  SampleTime=-1
  Data Store Write : DataStoreWrite  DataStoreName=adc_offset_ib_tmp  IndexOptions=Index vector (dialog)  Indices=1  OutputSizes=1
  Data Store Write1 : DataStoreWrite  DataStoreName=adc_offset_ic_tmp  IndexOptions=Index vector (dialog)  Indices=1  OutputSizes=1
  Data Store Write2 : DataStoreWrite  DataStoreName=cnt_calib  IndexOptions=Index vector (dialog)  Indices=1  OutputSizes=1
  Data Store Write3 : DataStoreWrite  DataStoreName=adc_offset_vc_tmp  IndexOptions=Index vector (dialog)  Indices=1  OutputSizes=1
  Data Store Write4 : DataStoreWrite  DataStoreName=adc_offset_ia_tmp  IndexOptions=Index vector (dialog)  Indices=1  OutputSizes=1
  Data Store Write5 : DataStoreWrite  DataStoreName=adc_offset_va_tmp  IndexOptions=Index vector (dialog)  Indices=1  OutputSizes=1
  Data Store Write6 : DataStoreWrite  DataStoreName=adc_offset_vb_tmp  IndexOptions=Index vector (dialog)  Indices=1  OutputSizes=1
  IIR Filter2 : Subsystem  Commented=on
  Subsystem1 : Subsystem
  Subsystem2 : Subsystem
  Subsystem3 : Subsystem
  Subsystem4 : Subsystem
  Subsystem5 : Subsystem
  Subsystem6 : Subsystem
  calib_ok : Outport
  wires:
  cnt_calib/1 -> Add/1
  Add/1 -> Data Store Write2/1
  Constant1/1 -> calib_ok/1
  Subsystem2/1(average) -> Data Store Write/1  "va"
  Constant/1 -> Add/2
  Subsystem1/1(average) -> Data Store Write1/1  "va"
  Subsystem3/1(average) -> Data Store Write4/1  "va"
  Subsystem4/1(average) -> Data Store Write3/1  "va"
  Subsystem6/1(average) -> Data Store Write5/1  "va"
  van/1 -> Subsystem6/1(sample)
  Subsystem5/1(average) -> Data Store Write6/1  "va"
  vcn/1 -> Subsystem4/1(sample)
  vbn/1 -> Subsystem5/1(sample)
  ia/1 -> Subsystem3/1(sample)
  ic/1 -> Subsystem1/1(sample)
  ib/1 -> Subsystem2/1(sample)

== system npc_controller/CONTROL/STATE-MACHINE/CPU_CONTROL_100_inv/updateCalib/done ==
  Action Port : ActionPort
  AUTO-CALIB_DONE : Subsystem
  CLEAR_FAULTS : Subsystem
  Function-Call Generator : simulink/Ports & Subsystems/Function-Call Generator  sample_time=-1  numberOfIterations=1  DisallowWideOutput=off
  Function-Call Split1 : FunctionCallSplit  NumOutputPorts=2
  Function-Call Split2 : FunctionCallSplit  NumOutputPorts=2
  RESET_TZ : Subsystem
  calib_ok : Outport
  wires:
  Function-Call Generator/1 -> Function-Call Split1/1
  Function-Call Split1/2 -> Function-Call Split2/1
  AUTO-CALIB_DONE/1(Out1) -> calib_ok/1
  Function-Call Split1/1 -> AUTO-CALIB_DONE/Trigger
  Function-Call Split2/1 -> RESET_TZ/Trigger
  Function-Call Split2/2 -> CLEAR_FAULTS/Trigger

== system npc_controller/CONTROL/STATE-MACHINE/CPU_CONTROL_100_inv/updatePll3p/PLL ==
  abc : Inport
  Demux : Demux  Commented=on  Outputs=3
  If1 : If  Commented=on  IfExpression=(u1 > 0)  ShowElse=off
  SRF_PLL : Subsystem
  Subsystem : Subsystem  Commented=on
  theta : Outport  OutDataTypeStr=single
  wires:
  SRF_PLL/3(theta) -> theta/1
  Subsystem/1(Out1) -> If1/1
  abc/1 -> SRF_PLL/1(Vabc), Demux/1
  Demux/1 -> Subsystem/1(In1)

== system npc_controller/CONTROL/STATE-MACHINE/CPU_CONTROL_100_inv/updateSequencePhA/pol_final1 ==
  vxn : Inport
  ix : Inport  Port=2
  Trigger : TriggerPort  TriggerType=function-call  VariantControl=(inherit)  PortDimensions=1
  If : If  NumInputs=2  IfExpression="((u1 == 1)  & (u2 == 2)) | ((u1 == 2)  & (u2 == 1))"
  Merge : Merge
  pol_vxn : Subsystem  TreatAsAtomicUnit=on
  prot : Subsystem  TreatAsAtomicUnit=on
  pol : Outport
  wires:
  ix/1 -> If/2
  vxn/1 -> pol_vxn/1(vxn), If/1
  Merge/1 -> pol/1
  If/2 -> pol_vxn/Action
  prot/1(Out1) -> Merge/1
  If/1 -> prot/Action
  pol_vxn/1(Out1) -> Merge/2

== system npc_controller/CONTROL/STATE-MACHINE/CPU_CONTROL_100_inv/updateSequencePhA/pol_ix1 ==
  note: 75dig -> 3iac
  ix : Inport
  Trigger : TriggerPort  TriggerType=function-call  VariantControl=(inherit)  PortDimensions=1
  If : If  IfExpression="(u1 > -8)  & (u1 < 8)"  ElseIfExpressions=u1 >= 8
  Merge : Merge  Inputs=3
  neg : Subsystem  TreatAsAtomicUnit=on
  pos : Subsystem  TreatAsAtomicUnit=on
  zero : Subsystem  TreatAsAtomicUnit=on
  pol_ix : Outport
  wires:
  ix/1 -> If/1
  If/1 -> zero/Action
  zero/1(Out1) -> Merge/1
  If/2 -> pos/Action
  If/3 -> neg/Action
  neg/1(Out1) -> Merge/3
  pos/1(Out1) -> Merge/2
  Merge/1 -> pol_ix/1

== system npc_controller/CONTROL/STATE-MACHINE/CPU_CONTROL_100_inv/updateSequencePhA/pol_vxn1 ==
  note: 16dig -> 5vac
  vxn : Inport
  ixn1 : Inport  Port=2
  Trigger : TriggerPort  TriggerType=function-call  VariantControl=(inherit)  PortDimensions=1
  Constant1 : Constant  Commented=on  Value=2048  OutDataTypeStr=single  SampleTime=-1
  If : If  IfExpression="(u1 > -16)  & (u1 < 16)"  ElseIfExpressions=u1 >= 16
  Merge : Merge  Inputs=3
  Sum1 : Sum  Commented=on  Inputs=|++
  neg : Subsystem  TreatAsAtomicUnit=on
  pos : Subsystem  TreatAsAtomicUnit=on
  zero : Subsystem  TreatAsAtomicUnit=on
  pol_vxn : Outport
  wires:
  Constant1/1 -> Sum1/2
  Sum1/1 -> ?
  vxn/1 -> If/1, Sum1/1
  ixn1/1 -> pos/1(ixn), neg/1(ixn)
  Merge/1 -> pol_vxn/1
  pos/1(Out1) -> Merge/2
  neg/1(Out1) -> Merge/3
  If/3 -> neg/Action
  If/2 -> pos/Action
  zero/1(Out1) -> Merge/1
  If/1 -> zero/Action

== system npc_controller/CONTROL/STATE-MACHINE/CPU_CONTROL_100_inv/updateSequencePhA/pol_vxn2 ==
  note: 16dig -> 5vac
  vxn : Inport
  Trigger : TriggerPort  TriggerType=function-call  VariantControl=(inherit)  PortDimensions=1
  If : If  IfExpression="(u1 > -16)  & (u1 < 16)"  ElseIfExpressions=u1 >= 16
  Merge : Merge  Inputs=3
  neg : Subsystem  TreatAsAtomicUnit=on
  pos : Subsystem  TreatAsAtomicUnit=on
  zero : Subsystem  TreatAsAtomicUnit=on
  pol_vxn : Outport
  wires:
  vxn/1 -> If/1
  If/1 -> zero/Action
  zero/1(Out1) -> Merge/1
  If/2 -> pos/Action
  If/3 -> neg/Action
  neg/1(Out1) -> Merge/3
  pos/1(Out1) -> Merge/2
  Merge/1 -> pol_vxn/1

== system npc_controller/CONTROL/STATE-MACHINE/CPU_CONTROL_100_inv/updateSequencePhA1/pol_final1 ==
  vxn : Inport
  ix : Inport  Port=2
  Trigger : TriggerPort  TriggerType=function-call  VariantControl=(inherit)  PortDimensions=1
  If : If  NumInputs=2  IfExpression="((u1 == 1)  & (u2 == 2)) | ((u1 == 2)  & (u2 == 1))"
  Merge : Merge
  pol_vxn : Subsystem  TreatAsAtomicUnit=on
  prot : Subsystem  TreatAsAtomicUnit=on
  pol : Outport
  wires:
  ix/1 -> If/2
  vxn/1 -> pol_vxn/1(vxn), If/1
  Merge/1 -> pol/1
  If/2 -> pol_vxn/Action
  prot/1(Out1) -> Merge/1
  If/1 -> prot/Action
  pol_vxn/1(Out1) -> Merge/2
